simulink model "csws_simulink_model"  (R2021a)
settings: Solver=FixedStepAuto  StartTime=0.0  StopTime=15  RelTol=1e-3
model workspace (MAT data in the model file):
  t = 0
libraries: simulink x1
(part 2 of 2)

== matlab function csws_simulink_model/Compute Function1 ==
  data: latitude input; longitude input; output output; speed input; time input; onlineData input; predictionTime input; maximumLateralAcceleration input; upperSafeLimit input; lowerRadius input; upperRadius input
function output = csws(latitude,longitude,speed,time,onlineData,predictionTime,maximumLateralAcceleration,upperSafeLimit,lowerRadius,upperRadius)
coder.extrinsic('plot');
coder.extrinsic('legend');
coder.extrinsic('audioread');
coder.extrinsic('audioplayer');
coder.extrinsic('serialport');
coder.extrinsic('readline');
coder.extrinsic('nmeaParser');
coder.extrinsic('getfield');
coder.extrinsic('set_param');

% coder.varsize('output');

[y, Fs] = audioread('alert.mp3');
player = audioplayer(y, Fs);

if(onlineData == 0)
    
        index = 3;

        data = [latitude(:) longitude(:) speed(:) time(:)];

        if ismember(-199, data)
            output = 0;
            return;
        end

        data = convertDataArray(data);

        allData = [data(index - 2,1) data(index - 2,2) data(index - 2,3); 
            data(index - 1,1) data(index - 1,2) data(index - 1,3); 
            data(index,1) data(index,2) data(index,3)
            ];
        predictedData = [data(index,1) data(index,2) data(index,3)];

        temp_data = [
            data(length(data(:,1))-2,1) data(length(data(:,1))-2,2) data(length(data(:,1))-2,3);
            data(length(data(:,1))-1,1) data(length(data(:,1))-1,2) data(length(data(:,1))-1,3); 
            data(length(data(:,1)),1) data(length(data(:,1)),2) data(length(data(:,1)),3)
            ];

        % predict coordinates
        for time = 1:predictionTime
            [predictedX, predictedY] = predictCoordinates(temp_data, 3, 1);  

            temp_data = [temp_data(2,1) temp_data(2,2) temp_data(2,3);
                temp_data(3,1) temp_data(3,2) temp_data(3,3);
                predictedX predictedY getNextSpeed(temp_data, 3);
                ];

            allData = [allData; [temp_data(3,1) temp_data(3,2) temp_data(3,3)]];
            predictedData = [predictedData; [temp_data(3,1) temp_data(3,2) temp_data(3,3)]];
        end
    % maximumLateralAcceleration
        allData = computeCurvatureRadiusAndSpeed(allData,maximumLateralAcceleration*upperSafeLimit/100);

        N = size(allData,1);
        allData = [allData,zeros(N,1)];

        allData = checkCurvatureRadiusAndSpeed(allData, lowerRadius, upperRadius);
        
        if ismember(1, allData(7,:))
            output = 1;
        else
            output = 0;
        end
        

%         xlim([-150 150])
%         ylim([-150 150])


        plot(allData(:,1), allData(:,2), 'b-o', 'DisplayName','referenced coordinates')
        hold on
        plot(predictedData(:,1), predictedData(:,2), 'g-o', 'DisplayName','predicted coordinates')
        plot(predictedData(1,1), predictedData(1,2), 'b-o')
        legend('referenced coordinates','predicted coordinates')

        if ismember(1, allData(:,7))
            set(gca, 'Color',[1 0 0])
%             playblocking(player); 
%             playblocking(player); 
        else
            set(gca, 'Color',[1 1 1])
        end

        hold off
else
        PORT = "COM15";
        device = serialport(PORT,9600)
        pnmea = nmeaParser("MessageIDs", "RMC");
        
        record = readline(device);
        
        while (isempty(record) || ~startsWith(record,'$GPRMC'))
            record = readline(device);
        end        
        
        nvm = pnmea(record);
        Latitude = getfield(nvm,'Latitude');
        Longitude = getfield(nvm,'Longitude');
        Speed = getfield(nvm,'GroundSpeed');
        Time = getfield(nvm,'UTCDateTime');
%         fldnm = 'Status';
%         nx2 = nvm.parameters.(fldnm)
%         latit = output(Latitude)
%         gpsData = struct('Latitude',output.Latitude,'Longitude',output.Longitude,'Speed',output.GroundSpeed,'Time',output.UTCDateTime,'Status',output.Status);


%     if (speed(3) > 21)
%         output = 1
%     else
%         output = 0
%     end


        output = 3
    end

end

%% compute radius of curvature and recommended speed

function [predictedData] = computeCurvatureRadiusAndSpeed(predictedData,safeLimitOfLateralAcceleration)
%     Alateral_max = 5.9 * 0.7;
    Alateral_max = safeLimitOfLateralAcceleration;

    [pathdistance,R,~] = curvature([predictedData(:,1) predictedData(:,2)]);
    predictedData = [predictedData pathdistance R];
    predictedData = [predictedData sqrt(predictedData(:, 5) * Alateral_max)];
end


%% reference to: https://uk.mathworks.com/matlabcentral/fileexchange/69452-curvature-of-a-1d-curve-in-a-2d-or-3d-space 

function [L,R,k] = curvature(input)
% Radius of curvature and curvature vector for 2D or 3D curve
%  [L,R,k] = curvature(X)
%   X:   2 or 3 column array of x, y (and possibly z) coordiates
%   L:   Cumulative arc length
%   R:   Radius of curvature
%   k:   Curvature vector
% The scalar curvature value is 1./R
% Version 2.6: Calculates end point values for closed curve
%   fefefe = X

  coder.varsize('X');
  coder.varsize('L');
  coder.varsize('R');
  coder.varsize('k');
  X = input;

  N = size(X,1);
  dims = size(X,2);
  if dims == 2
    X = [X,zeros(N,1)];  % Use 3D expressions for 2D as well
  end
  L = zeros(N,1);
  R = NaN(N,1);
  k = NaN(N,3);
  for i = 2:N-1
    [R(i),~,k(i,:)] = circumcenter(X(i,:)',X(i-1,:)',X(i+1,:)');
    L(i) = L(i-1)+norm(X(i,:)-X(i-1,:));
  end
  if norm(X(1,:)-X(end,:)) < 1e-10 % Closed curve. 
    [R(1),~,k(1,:)] = circumcenter(X(end-1,:)',X(1,:)',X(2,:)');
    R(end) = R(1);
    k(end,:) = k(1,:);
    L(end) = L(end-1) + norm(X(end,:)-X(end-1,:));
  end
  i = N;
  L(i) = L(i-1)+norm(X(i,:)-X(i-1,:));
  if dims == 2
    k = k(:,1:2);
  end
end

%% reference to: https://uk.mathworks.com/matlabcentral/fileexchange/69452-curvature-of-a-1d-curve-in-a-2d-or-3d-space 

function [R,M,k] = circumcenter(A,B,C)
% Center and radius of the circumscribed circle for the triangle ABC
%  A,B,C  3D coordinate vectors for the triangle corners
%  R      Radius
%  M      3D coordinate vector for the center
%  k      Vector of length 1/R in the direction from A towards M
%         (Curvature vector)
  D = cross(B-A,C-A);
  b = norm(A-C);
  c = norm(A-B);
  if nargout == 1
    a = norm(B-C);     % slightly faster if only R is required
    R = a*b*c/2/norm(D);
    if norm(D) == 0
      R = Inf;
    end
    return
  end
  E = cross(D,B-A);
  F = cross(D,C-A); 
  G = (b^2*E-c^2*F)/norm(D)^2/2;
  M = A + G;
  R = norm(G);  % Radius of curvature
  if R == 0
    k = G;
  elseif norm(D) == 0
    R = Inf;
    k = D;
  else
    k = G'/R^2;   % Curvature vector
  end
end

%% check if radius of curvature is valid and actual speed is higher than recommended

function [predictedData] = checkCurvatureRadiusAndSpeed(predictedData,lowerRadius,upperRadius)
    Rmin = lowerRadius;
    Rmax = upperRadius;
    
    for k=1:size(predictedData,1)
        if predictedData(k,5) < Rmin || predictedData(k,5) > Rmax
            predictedData(k,7) = 0;
        else
            if predictedData(k,3) > predictedData(k,6)
                predictedData(k,7) = 1;
            else
                predictedData(k,7) = 0;
            end
        end
    end
end

%% compute angle between coordinates

function next_angle = computeCoordinateAngle(data, index, time)
    prev_angle = atan2( (data(index - 1,2) - data(index - 2,2)) , (data(index - 1,1) - data(index - 2,1)));
    act_angle = atan2( (data(index,2) - data(index - 1,2)) , (data(index,1) - data(index - 1,1)));
    
    next_angle = act_angle + time*(act_angle - prev_angle);
end

%% convert latitude, longitude to cartesian coordinate system

function [data] = convertDataArray(data)
    coder.extrinsic('latlon2local');
    [xCoordinate, yCoordinate] = latlon2local(data(:,1), data(:,2), 0, [data(1,1), data(1,2), 0]);
    data = [xCoordinate yCoordinate data(:,3) data(:,4)];

%     xBegin = data(1,1)
%     yBegin = data(1,2)
%     
%     [xCoordinates,yCoordinates]=latlon2xy(data(1,1),data(1,2),xBegin,yBegin,'sphere');
%     [xCoordinates2,yCoordinates2]=latlon2xy(data(2,1),data(2,2),xBegin,yBegin,'sphere');
%     [xCoordinates3,yCoordinates3]=latlon2xy(data(3,1),data(3,2),xBegin,yBegin,'sphere');
% 
%     fe = [xCoordinates yCoordinates data(1,3) data(1,4); 
%         xCoordinates2,yCoordinates2 data(2,3) data(2,4); 
%         xCoordinates3,yCoordinates3 data(3,3) data(3,4); 
%     ];
% 
%     data = fe

%     [xCoordinate, yCoordinate] = latlon2local(data(:,1), data(:,2), 0, [data(1,1), data(1,2), 0]);
%     [xCoordinate, yCoordinate] = latlon2xy(data(:,1),data(:,2),data(1,1), data(1,2),'sphere');
%     latlon2xy(data(:,1),data(:,2),data(1,1), data(1,2),'sphere');
%     data = [xCoordinate yCoordinate data(:,3) data(:,4)];
end

%% get speed of last referenced point for predicted points

function [nextspeed] = getNextSpeed(data, index)
    nextspeed = data(index,3);
    if nextspeed < 0
        nextspeed = 0;
    end
end

%% insert GPS data to data structure
function [predictedX,predictedY] = predictCoordinates(data, index, time)
    speed = getNextSpeed(data, index);
    next_angle = computeCoordinateAngle(data, index, time);
% 
    predictedX = predictCoordinateX(data, index, next_angle, time, speed);
    predictedY = predictCoordinateY(data, index, next_angle, time, speed);
end

%% predict x coordinate

function predictedX = predictCoordinateX(data, index, angle, time, speed)
    predictedX = data(index,1) + speed * time * cos(angle);
end

%% predict y coordinate

function predictedY = predictCoordinateY(data, index, angle, time, speed)
    predictedY = data(index,2) + speed * time * sin(angle);
end

%%





% ----------------
% function predX = getX(lon)
% %     double x = fmod((width*(180+lon)/360), (width +(width/2)));
%     x = lon * pi * 6378137 / 180;
%     predX = x
% 
% %     return x;
% end
% 
% function predY = getY(lat)
% %     double x = fmod((width*(180+lon)/360), (width +(width/2)));
% 
%     y = log(tan((90 + lat) * pi / 360)) / (pi / 180)
% %     var y = Math.Log(Math.Tan((90 + lat) * Math.PI / 360)) / (Math.PI / 180);
%     y = y * pi * 6378137 / 180;
%     predY = y
% 
% %     return x;
% end
% 
% 
% % double testClass::getY(double lat, int height, int width)
% % {
% %     // height and width are map height and width
% %     double PI = 3.14159265359;
% %     double latRad = lat*PI/180;
% % 
% %     // get y value
% %     double mercN = log(tan((PI/4)+(latRad/2)));
% %     double y     = (height/2)-(width*mercN/(2*PI));
% %     return y;
% % }
% 
% function m = fmod(a, b)
% 
%     % Where the mod function returns a value in region [0, b), this
%     % function returns a value in the region [-b, b), with a negative
%     % value only when a is negative.
% 
%     if a == 0
%         m = 0;
%     else
%         m = mod(a, b) + (b*(sign(a) - 1)/2);
%     end
% 
% end
% 
% 
% % data = convertDataArray(workdata);
% 
% % x = workdata(:,1)
% % f = workdata(:,2)
% 
% 
% % y = abs(-5);
% % data = workdata
% % [xCoordinate, yCoordinate] = latlon2local(data(:,1), data(:,2), 0, [data(1,1), data(1,2), 0]);
% % y = [xCoordinate, yCoordinate]
% % y = [u(1) u(2) u(3) u(4) u(5) u(6) u(7) u(8) u(9) u(10) u(11) u(12)];
% 
% % function output = latlon2xy(latitude, longitude)
% %     latitude = 2
% %     longitude = 3
% %     output = 4
% % end
% -----------------------


%% reference to https://github.com/ashao/matlab/blob/master/external/jlab/latlon2xy.m
function[x,y,d]=latlon2xy(varargin)
% LATLON2XY  Converts latitude and longitude into local Cartesian coordinates.
%
%   [X,Y]=LATLON2XY(LAT,LON,LATO,LONO) converts (LAT,LON) with units
%   of degrees into displacements (X,Y) in a plane tangent to the 
%   earth at the point (LATO, LONO). X and Y have units of kilometers.
%
%   CX=LATLON2XY(LAT,LON,LATO,LONO) with one output argument returns 
%   the location as a complex-valued quantity X+SQRT(-1)*Y. NANs in
%   LAT or LON become NAN+SQRT(-1)*NAN.
%   
%   LAT and LON are arrays of the same size.  LATO and LONO are either
%   also arrays of this size, or else scalars.  X and Y have the same
%   size as the input arrays.  
%
%   X and Y are computed by projecting the tangent plane onto the 
%   sphere using full spherical geometry.  
%
%   The radius of the earth is given by the function RADEARTH.
%
%   Note that X and Y are set to NANs for points on the opposite side
%   of the earth from the tangent plane, that is, where the great 
%   circle distance would exceed RADEARTH * pi/2.  
%   ___________________________________________________________________
%
%   Great circle distance
%
%   [X,Y,D]=LATLON2XY(...) also returns the great circle distance D
%   between the two sets of points.  
%
%   For points on the same side on the earth from the tangent plane,
%   i.e. where the great circle distance is less than RADEARTH * pi/2,
%   LATLON2XY gives the same distance as SPHEREDIST.  
%
%   However, for points on the opposite side of the earth, LATLON2XY
%   returns NANs whereas SPHEREDIST returns the correct distance.
%
%   The great circle distance computed here is useful because it is 
%   a fast computation if X and Y are already known.
%   ___________________________________________________________________
%
%   Cell array input / output
%
%   LATLON2XY returns cell array output given cell array input.  
%
%   That is, if LAT, LON, LATO, and LONO are all cell arrays of length K, 
%   containing K different numerical arrays, then the output will also be 
%   cell arrays of length K.  
%   ___________________________________________________________________
%
%   Complex-valued input / output
%
%   If LON and LAT are complex-valued, the real and imaginary parts are 
%   converted separately to give complex-valued X and complex-valued Y.  
%   ___________________________________________________________________
%
%   LATLON2XY is inverted by XY2LATLON.
%
%   See also XY2LATLON, LATLON2UV, SPHEREDIST.
%
%   Usage:  [x,y]=latlon2xy(lat,lon,lato,lono);
%           cx=latlon2xy(lat,lon,lato,lono);
%
%   'latlon2xy --t' runs some tests.
%   _________________________________________________________________
%   This is part of JLAB --- type 'help jlab' for more information
%   (C) 2000--2011 J.M. Lilly --- type 'help jlab_license' for details        
  
    if strcmp(varargin{1}, '--t')
      latlon2xy_test,return
    end

    na=nargin;
    if ischar(varargin{end})
        str=varargin{end};
        na=na-1;
    else 
        str='sphere';
    end


    lat=varargin{1};
    lon=varargin{2};
    lato=varargin{3};
    lono=varargin{4};

    R=6378137;

    if ~iscell(lat)
        if isreal(lat)
            [x,y,d]=latlon2xy_celloop(nargout,lat,lon,lato,lono,R,str);
        else
            [xr,yr,dr]=latlon2xy_celloop(nargout,real(lat),real(lon),lato,lono,R,str);
            [xi,yi,di]=latlon2xy_celloop(nargout,imag(lat),imag(lon),lato,lono,R,str);
            x=xr+sqrt(-1)*xi;
            y=yr+sqrt(-1)*yi;
            d=dr+sqrt(-1)*di;
        end
    else
        for i=1:length(lat)
            if isreal(lat{i})
                [x{i},y{i},d{i}]=latlon2xy_celloop(nargout,lat{i},lon{i},lato{i},lono{i},R,str);
            else
               [xr,yr,dr]=latlon2xy_celloop(nargout,real(lat{i}),real(lon{i}),lato{i},lono{i},R,str);
               [xi,yi,di]=latlon2xy_celloop(nargout,imag(lat{i}),imag(lon{i}),lato{i},lono{i},R,str);
               x{i}=xr+sqrt(-1)*xi;
               y{i}=yr+sqrt(-1)*yi;
               d{i}=dr+sqrt(-1)*di;
            end  
        end
    end
end

function[x,y,d]=latlon2xy_celloop(N,lat,lon,lato,lono,R,str)
    d=[];
    if numel(lato)==1
        lato=lato+0*lat;
    end
    if numel(lono)==1
        lono=lono+0*lat;
    end

    if strcmp(str(1:3),'sma')
         [x,y]=latlon2xy_cartesian(lat,lon-lono,lato,R);
    elseif strcmp(str(1:3),'sph')
         if N<3
            [x,y]=latlon2xy_sphere(lat,lon-lono,lato,R);
         else
            [x,y,d]=latlon2xy_sphere(lat,lon-lono,lato,R);
         end
    end

    if N==1 
      x=real(x)+sqrt(-1)*real(y);
      index=find(isnan(real(x))|isnan(imag(x)));
      if ~isempty(index)
         x(index)=nan+sqrt(-1)*nan;
      end
    end
    end

    function[x,y]=latlon2xy_cartesian(lat,lon,lato,R)

    [lat,lon,lato]=jdeg2rad(lat,lon,lato);
    r1=R.*cos(lato);
    dlon=angle(rot(lon));
    x=dlon.*r1;
    y=(lat-lato).*R;
end

function[x,y,d]=latlon2xy_sphere(lat,lon,lato,R)
    x=nan*lat;
    y=nan*lon;

    %  Check to see if I'm in the same hemisphere, or on the other side
    %  Here I'm implementing latlon2xyz to find dot product of two vectors
    %  and, I avoid recomputing angles

    %if ~isreal(lato),lato,end
    coslat=cosd(lat);
    coslon=cosd(lon);
    coslato=cosd(lato);
    sinlato=sind(lato);
    sinlat=sind(lat);

    %  The next line is the dot product, i.e. x.*x2+z.*z2 with
    %  x=cos(lat).*cos(lon);z=sin(lat);
    %  x2=cos(lato);z2=sin(lato);

    index=find(coslat.*coslon.*coslato+sinlato.*sinlat>0);

    %  Now implement these equations
    %    x=R*cos(lat).*sin(lon);
    %    y=-R*cos(lat).*sin(lato).*cos(lon)+R.*cos(lato).*sin(lat);
    %  but only for points in the same hemisphere.

    %  To derive these equations, calculate the xyz position in space of both 
    %  a lat/lon point, and a point on the tangent plane.  It's helpful to
    %  define d(x,y)=perpendicular distance to Earth from tangent plane 
    %  where  d(x,y)=R - sqrt(R.^2-x^2-y^2)

    %  Also note, correctly, that y>0 at the north pole for delta lon=180 
    %                         but y>0 at the south pole for delta lon=0;

    if ~isempty(index)
        x(index)=R*coslat(index).*sind(lon(index));
        y(index)=-R*coslat(index).*sinlato(index).*coslon(index)+R.*coslato(index).*sinlat(index);
    end

    %d=2*R.*asin(frac(1,sqrt(2)).*sqrt(1-sqrt(1-frac(x.^2+y.^2,R.^2)))); 
    if nargout==3
        if ~isempty(index)
            d=nan*lon;
            d(index)=2*R.*asin(frac(1,sqrt(2)).*sqrt(1-sqrt(1-frac(x(index).^2+y(index).^2,R.^2)))); 
        end
    end
end

== matlab function csws_simulink_model/MATLAB Function5 ==
  data: latitude output; longitude output; speed output
function [latitude, longitude, speed] = GPSDataReceiver

coder.extrinsic('serialport');
coder.extrinsic('readline');
coder.extrinsic('nmeaParser');
coder.extrinsic('getfield');
coder.extrinsic('set_param');
coder.extrinsic('strings');
coder.extrinsic('strrep');

coder.extrinsic('str2double');
coder.extrinsic('get_param');
coder.extrinsic('gcb');
coder.extrinsic('append');

inputPort = get_param(gcb,'inputPort');

% coder.varsize('latitude')
% coder.varsize('longitude')
% coder.varsize('speed')
% coder.varsize('time')
latitude=zeros(1,1);
longitude=zeros(1,1);
speed=zeros(1,1);
% time=strings(1);

        PORT = append("COM",inputPort);
        device = serialport(PORT,9600);
        pnmea = nmeaParser("MessageIDs", "RMC");
        
        record = readline(device);
        
        while (isempty(record) || ~startsWith(record,'$GPRMC'))
            record = readline(device);
        end        
        
        nvm = pnmea(record);
        latitude = getfield(nvm,'Latitude');
        longitude = getfield(nvm,'Longitude');
        speed = getfield(nvm,'GroundSpeed');
        
        latitude = strrep(latitude,'.',',');
        longitude = strrep(longitude,'.',',');
        speed = strrep(speed,'.',',');
%         time = getfield(nvm,'UTCDateTime');

%         a = size(latitude)
%         b = size(fx)  
%         x = length(latitude)
%         b = size(latitude(1))
% [latitude, longitude, speed, time]
% y = latitude
% y = latitude
f = latitude

== matlab function csws_simulink_model/MATLAB Function1 ==
  data: lowerBound input; upperBound input
function checkCurvatureRadiusRange(lowerBound, upperBound)
    if(lowerBound < 0 || upperBound < 0)
        error('Negative values of curvature bound are not supported')
    end

    if(lowerBound <= upperBound)
        return
    else
        error('Lower bound of curvature radius must be smaller than upper bound')
    end

== matlab function csws_simulink_model/MATLAB Function2 ==
  data: latitude output; longitude output; speed output
function [latitude, longitude, speed] = GPSDataReceiver

coder.extrinsic('serialport');
coder.extrinsic('readline');
coder.extrinsic('nmeaParser');
coder.extrinsic('getfield');
coder.extrinsic('set_param');
coder.extrinsic('strings');
coder.extrinsic('strrep');

coder.extrinsic('str2double');
coder.extrinsic('get_param');
coder.extrinsic('gcb');
coder.extrinsic('append');

inputPort = get_param(gcb,'inputPort');

% coder.varsize('latitude')
% coder.varsize('longitude')
% coder.varsize('speed')
% coder.varsize('time')
latitude=zeros(1,1)
longitude=zeros(1,1)
speed=zeros(1,1)
% time=strings(1)

        PORT = append("COM",inputPort);
        device = serialport(PORT,4800);
        pnmea = nmeaParser("MessageIDs", "RMC");
        
        record = readline(device);
        
        while (isempty(record) || ~startsWith(record,'$GPRMC'))
            record = readline(device);
        end        
        
        nvm = pnmea(record);
        latitude = getfield(nvm,'Latitude');
        longitude = getfield(nvm,'Longitude');
        speed = getfield(nvm,'GroundSpeed');
        
        latitude = strrep(latitude,'.',',')
        longitude = strrep(longitude,'.',',')
        speed = strrep(speed,'.',',')
%         time = getfield(nvm,'UTCDateTime');

%         a = size(latitude)
%         b = size(fx)  
%         x = length(latitude)
%         b = size(latitude(1))
% [latitude, longitude, speed, time]
% y = latitude
% y = latitude
f = latitude

== matlab function csws_simulink_model/MATLAB Function3 ==
  data: a input; y output; b input; c input
function y = fcn(a,b,c)
    m = a
    n = b
    o = c
y = 5;

== matlab function csws_simulink_model/MATLAB Function6 ==
  data: a input; y output; b input; c input
function y = fcn(a,b,c)
    m = a
    n = b
    o = c
y = 5;

== matlab function csws_simulink_model/MATLAB Function4 ==
  data: latitude output; longitude output; speed output
function [latitude, longitude, speed] = fcn

coder.extrinsic('serialport');
coder.extrinsic('readline');
coder.extrinsic('nmeaParser');
coder.extrinsic('getfield');
coder.extrinsic('set_param');
coder.extrinsic('strings');
coder.extrinsic('strrep');

% coder.varsize('latitude')
% coder.varsize('longitude')
% coder.varsize('speed')
% coder.varsize('time')
latitude=zeros(1,1)
longitude=zeros(1,1)
speed=zeros(1,1)
% time=strings(1)

        PORT = "COM15";
        device = serialport(PORT,9600);
        pnmea = nmeaParser("MessageIDs", "RMC");
        
        record = readline(device);
        
        fx = 0
        
        while (isempty(record) || ~startsWith(record,'$GPRMC'))
            record = readline(device);
        end        
        
        nvm = pnmea(record);
        latitude = getfield(nvm,'Latitude');
        longitude = getfield(nvm,'Longitude');
        speed = getfield(nvm,'GroundSpeed');
        
        latitude = strrep(latitude,'.',',')
        longitude = strrep(longitude,'.',',')
        speed = strrep(speed,'.',',')
%         time = getfield(nvm,'UTCDateTime');

%         a = size(latitude)
%         b = size(fx)  
%         x = length(latitude)
%         b = size(latitude(1))
% [latitude, longitude, speed, time]
% y = latitude
% y = latitude
f = latitude
